simulink model "TV_full_CARSIM_24b"  (R2024b)
settings: Solver=FixedStepAuto  StartTime=0  StopTime=30  FixedStep=0.0005  RelTol=1e-3
undefined symbols (not defined in the file): DGain, FBgain, FFgain, g, GR, h, IGain, Iz, Kb, Kd, Ki, Kn, Kp, L, mu, Mz_dTm_convertion, NGain, PGain, s_desired, TC_switch, Tmax, TV_switch, vx_vector
libraries: slpidlib x2, Solver_SF x1, simulink x1
settings Model: Creator=savchenko.6  LastModifiedBy=account
settings DataIOCC: ReturnWorkspaceOutputs=off
settings RTWCC: GPUComputeCapability=3.5
settings ConfigComp: CovBoundaryAbsTol=1.0e-5

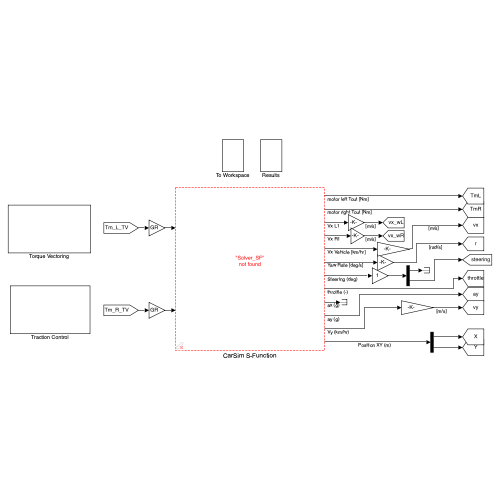
[thumbnail: Simulink's stored preview of the top-level diagram]
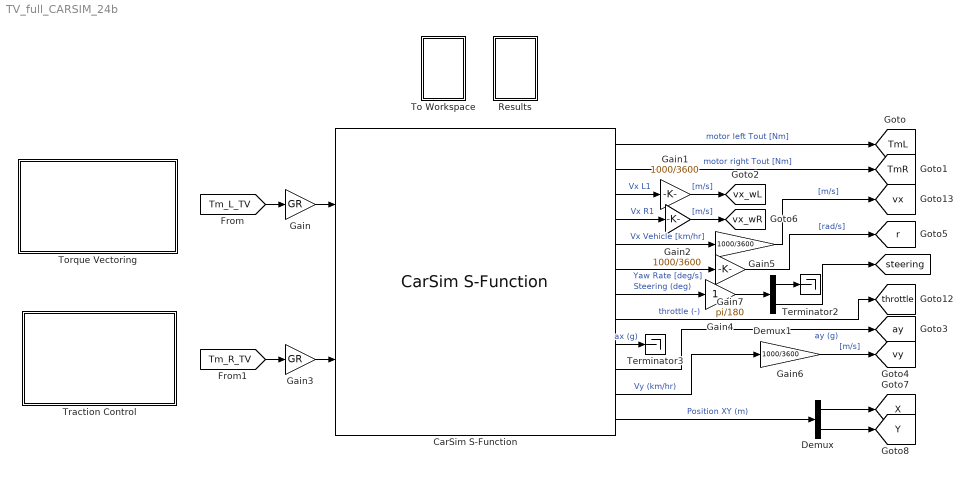
== system TV_full_CARSIM_24b ==
  CarSim S-Function : Solver_SF/CarSim S-Function  Priority=1  SIMFILE=simfile.sim  Run_RTs=off  vs_state_ind=Run  StopMode_ind=Vehicle Model
  Demux : Demux  Outputs=2
  Demux1 : Demux  Outputs=2
  Gain : Gain  Gain=GR
  Gain{1..2,5..6} (4 alike) : Gain  Gain=1000/3600
  Gain3 : Gain  Gain=GR
  Gain4 : Gain
  Gain7 : Gain  Gain=pi/180
  Results : Subsystem
  Terminator2 : Terminator
  Terminator3 : Terminator
  To Workspace : Subsystem
  Torque Vectoring : Subsystem
  Traction Control : Subsystem
  tag scope: TmL=global, TmR=global, X=global, Y=global, ay=global, r=global, steering=global, throttle=global, vx=global, vx_wL=global, vx_wR=global, vy=global
  wires:
  CarSim S-Function/5 -> Gain5/1  "Vx Vehicle [km/hr]"
  CarSim S-Function/10 -> [ay]  "ay (g)"
  CarSim S-Function/11 -> Gain6/1  "Vy (km/hr)"
  CarSim S-Function/6 -> Gain7/1  "Yaw Rate [deg/s]"
  CarSim S-Function/1 -> [TmL]  "motor left Tout [Nm]"
  CarSim S-Function/2 -> [TmR]  "motor right Tout [Nm]"
  CarSim S-Function/3 -> Gain1/1  "Vx L1"
  CarSim S-Function/4 -> Gain2/1  "Vx R1"
  CarSim S-Function/7 -> Gain4/1  "Steering (deg)"
  CarSim S-Function/8 -> [throttle]  "throttle (-)"
  CarSim S-Function/9 -> Terminator3/1  "ax (g)"
  CarSim S-Function/12 -> Demux/1  "Position XY (m)"
  Demux/1 -> [X]
  Demux/2 -> [Y]
  Gain7/1 -> [r]  "[rad/s]"
  Gain5/1 -> [vx]  "[m/s]"
  Demux1/1 -> Terminator2/1
  Gain1/1 -> [vx_wL]  "[m/s]"
  Gain2/1 -> [vx_wR]  "[m/s]"
  [Tm_R_TV] -> Gain3/1
  [Tm_L_TV] -> Gain/1
  Gain/1 -> CarSim S-Function/1
  Gain3/1 -> CarSim S-Function/2
  Gain4/1 -> Demux1/1
  Gain6/1 -> [vy]  "[m/s]"
  Demux1/2 -> [steering]

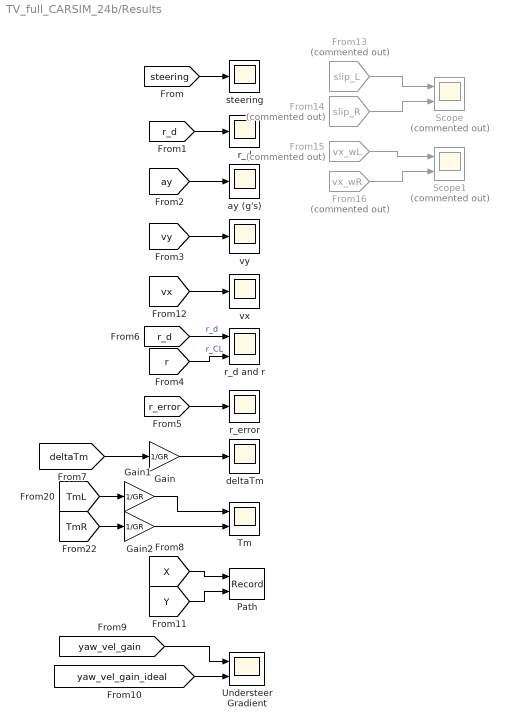
== system TV_full_CARSIM_24b/Results ==
  From13 : From  Commented=on  GotoTag=slip_L  TagVisibility=global
  From14 : From  Commented=on  GotoTag=slip_R  TagVisibility=global
  From15 : From  Commented=on  GotoTag=vx_wL  TagVisibility=global
  From16 : From  Commented=on  GotoTag=vx_wR  TagVisibility=global
  Gain : Gain  Gain=1/GR
  Gain1 : Gain  Gain=1/GR
  Gain2 : Gain  Gain=1/GR
  Path : Record  FileSettingsInternal="{\"entries\":[{\"content\":{\"excelSettings\":{\"content\":{},\"type\":\"Streamout.ExcelSettings\"},\"parquetSettings\":{\"content\":{},\"type\":\"Streamout.ParquetSettings\"}},\"type\":\"Streamout.FileSettingStorage\",\"uuid\":\"\"}],\"packageUris\":[\"http:\\/\\/schema.mathworks.com\\/mf0\\/streamout_blocks\\/R2020a\"],\"version\":\"1.0\"}"  Layout=[1 1]  SignalsInternal="{\"entries\":[{\"content\":{\"signals\":[{\"content\":{\"blockPath\":[],\"dimensions\":[1],\"domain\":\"\",\"lineColor\":\"#fe330a\",\"port\":1,\"signalID\":1,\"signalName\":\"From8\"},\"type\":\"RecordBlkView.Signal\",\"uuid\":\"\"},{\"content\":{\"blockPath\":[],\"dimensions\":[1],\"domain\":\"\",\"lineColor\":\"#22b573\",\"port\":2,\"signalID\":2,\"signalName\":\"From11\"},\"type\":\"RecordBlkView.Signal\",\"uuid\":\"\"}]},\"type\":\"RecordBlkView.InputSignals\",\"uuid\":\"\"}],\"packageUris\":[\"http:\\/\\/schema.mathworks.com\\/mf0\\/streamout_blocks\\/R2020a\"],\"version\":\"1.0\"}"  VisualizationBindings="{\"xyplotplugin\":{\"info\":[{\"series\":[],\"subplotID\":1}]}}"  CompatibilityTag=XY
  Scope : Scope  Commented=on  NumInputPorts=2
  Scope1 : Scope  Commented=on  NumInputPorts=2
  Tm : Scope  NumInputPorts=2
  Understeer Gradient : Scope  NumInputPorts=2
  ay (g's) : Scope
  deltaTm : Scope
  r_d : Scope
  r_d and r : Scope  NumInputPorts=2
  r_error : Scope
  steering : Scope
  vx : Scope
  vy : Scope
  wires:
  [deltaTm] -> Gain/1
  [r] -> r_d and r/2  "r_CL"
  [TmR] -> Gain2/1
  [steering] -> steering/1
  [Y] -> Path/2
  [vy] -> vy/1
  [TmL] -> Gain1/1
  [r_d] -> r_d and r/1  "r_d"
  [r_d] -> r_d/1
  [ay] -> ay (g's)/1
  [r_error] -> r_error/1
  [X] -> Path/1
  [yaw_vel_gain] -> Understeer Gradient/1
  [yaw_vel_gain_ideal] -> Understeer Gradient/2
  [vx] -> vx/1
  From13/1 -> Scope/1
  From14/1 -> Scope/2
  From15/1 -> Scope1/1
  From16/1 -> Scope1/2
  Gain/1 -> deltaTm/1
  Gain1/1 -> Tm/1
  Gain2/1 -> Tm/2

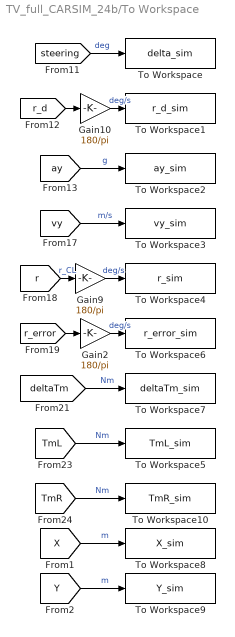
== system TV_full_CARSIM_24b/To Workspace ==
  Gain10 : Gain  Gain=180/pi
  Gain2 : Gain  Gain=180/pi
  Gain9 : Gain  Gain=180/pi
  To Workspace : ToWorkspace  VariableName=delta_sim  SampleTime=-1
  To Workspace1 : ToWorkspace  VariableName=r_d_sim  SampleTime=-1
  To Workspace10 : ToWorkspace  VariableName=TmR_sim  SampleTime=-1
  To Workspace2 : ToWorkspace  VariableName=ay_sim  SampleTime=-1
  To Workspace3 : ToWorkspace  VariableName=vy_sim  SampleTime=-1
  To Workspace4 : ToWorkspace  VariableName=r_sim  SampleTime=-1
  To Workspace5 : ToWorkspace  VariableName=TmL_sim  SampleTime=-1
  To Workspace6 : ToWorkspace  VariableName=r_error_sim  SampleTime=-1
  To Workspace7 : ToWorkspace  VariableName=deltaTm_sim  SampleTime=-1
  To Workspace8 : ToWorkspace  VariableName=X_sim  SampleTime=-1
  To Workspace9 : ToWorkspace  VariableName=Y_sim  SampleTime=-1
  wires:
  [vy] -> To Workspace3/1  "m/s"
  [ay] -> To Workspace2/1  "g"
  Gain10/1 -> To Workspace1/1  "deg/s"
  [deltaTm] -> To Workspace7/1  "Nm"
  Gain2/1 -> To Workspace6/1  "deg/s"
  [TmR] -> To Workspace10/1  "Nm"
  [r] -> Gain9/1  "r_CL"
  [steering] -> To Workspace/1  "deg"
  [r_d] -> Gain10/1
  [TmL] -> To Workspace5/1  "Nm"
  [r_error] -> Gain2/1
  Gain9/1 -> To Workspace4/1  "deg/s"
  [X] -> To Workspace8/1  "m"
  [Y] -> To Workspace9/1  "m"

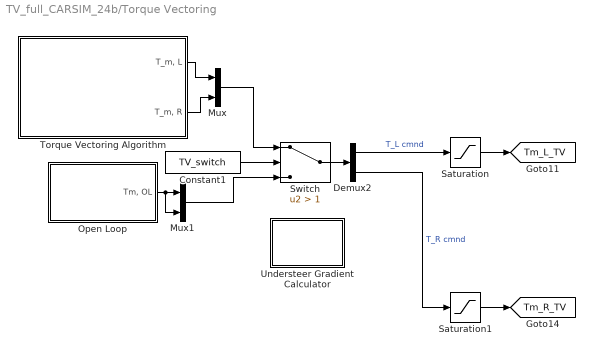
== system TV_full_CARSIM_24b/Torque Vectoring ==
  Constant1 : Constant  Value=TV_switch
  Demux2 : Demux  Outputs=2
  Mux : Mux  Inputs=2
  Mux1 : Mux  Inputs=2
  Open Loop : Subsystem
  Saturation : Saturate  UpperLimit=Tmax  LowerLimit=0
  Saturation1 : Saturate  UpperLimit=Tmax  LowerLimit=0
  Switch : Switch  Criteria=u2 > Threshold  Threshold=1  SaturateOnIntegerOverflow=off  InputSameDT=off
  Torque Vectoring Algorithm : Subsystem
  Understeer Gradient Calculator : Subsystem
  tag scope: Tm_L_TV=global, Tm_R_TV=global
  wires:
  Demux2/2 -> Saturation1/1  "T_R cmnd"
  Mux/1 -> Switch/1
  Constant1/1 -> Switch/2
  Torque Vectoring Algorithm/2("T_m, R") -> Mux/2
  Demux2/1 -> Saturation/1  "T_L cmnd"
  Open Loop/1("Tm, OL") -> Mux1/2, Mux1/1
  Torque Vectoring Algorithm/1("T_m, L") -> Mux/1
  Mux1/1 -> Switch/3
  Switch/1 -> Demux2/1
  Saturation/1 -> [Tm_L_TV]
  Saturation1/1 -> [Tm_R_TV]

== system TV_full_CARSIM_24b/Traction Control ==
  Trcation Control Algorithm : Subsystem
  tag scope: Tm_L_TC=global, Tm_R_TC=global, slip=global, slip_L=global, slip_R=global
  wires:
  [Tm_R_TV] -> Trcation Control Algorithm/5(Tm_R_TV)
  Trcation Control Algorithm/3(Tm_R_TC) -> [Tm_R_TC]
  [vx_wL] -> Trcation Control Algorithm/2(vx_wL)
  Trcation Control Algorithm/1(slip_L) -> [slip_L]
  Trcation Control Algorithm/4(Tm_L_TC) -> [Tm_L_TC]
  Trcation Control Algorithm/2(slip_R) -> [slip_R]
  [Tm_L_TV] -> Trcation Control Algorithm/4(Tm_L_TV)
  [vx_wR] -> Trcation Control Algorithm/3(vx_wR)
  [vx] -> Trcation Control Algorithm/1(vx)
  Trcation Control Algorithm/5(slip) -> [slip]

== system TV_full_CARSIM_24b/Torque Vectoring/Open Loop ==
  Gain : Gain  Gain=21
  "Tm, OL" : Outport
  wires:
  [throttle] -> Gain/1
  Gain/1 -> "Tm, OL"/1

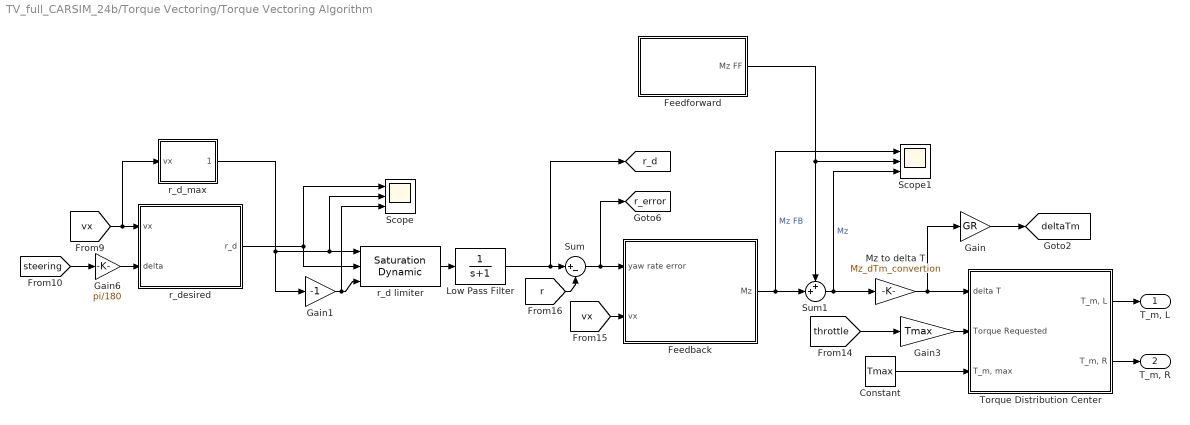
== system TV_full_CARSIM_24b/Torque Vectoring/Torque Vectoring Algorithm ==
  Constant : Constant  Value=Tmax
  Feedback : Subsystem
  Feedforward : Subsystem
  Gain : Gain  Gain=GR
  Gain1 : Gain  Gain=-1
  Gain3 : Gain  Gain=Tmax
  Gain6 : Gain  Gain=pi/180
  Low Pass Filter : TransferFcn  Denominator=[1 1]
  Mz to delta T : Gain  Gain=Mz_dTm_convertion
  Scope : Scope  NumInputPorts=3
  Scope1 : Scope  NumInputPorts=3
  Sum : Sum  Inputs=|+-
  Sum1 : Sum  Inputs=++|
  Torque Distribution Center : Subsystem
  r_d limiter : simulink/Discontinuities/Saturation Dynamic  OutMin=[]  OutMax=[]  OutDataTypeStr=Inherit: Same as second input  OutDataType=fixdt(1, 16)  OutScaling=2^-10  RndMeth=Round  DoSatur=off
  r_d_max : Subsystem
  r_desired : Subsystem
  "T_m, L" : Outport
  "T_m, R" : Outport  Port=2
  tag scope: deltaTm=global, r_d=global, r_error=global
  wires:
  r_d_max/1(r_d_max) -> Scope/2, r_d limiter/1, Gain1/1
  Sum/1 -> Feedback/1(yaw rate error), [r_error]
  r_desired/1(r_d) -> r_d limiter/2, Scope/1
  Gain3/1 -> Torque Distribution Center/2(Torque Requested)
  [r] -> Sum/2
  [steering] -> Gain6/1
  Gain1/1 -> Scope/3, r_d limiter/3
  [throttle] -> Gain3/1
  [vx] -> r_d_max/1(vx), r_desired/1(vx)
  Mz to delta T/1 -> Torque Distribution Center/1(delta T), Gain/1
  Gain6/1 -> r_desired/2(delta)
  Constant/1 -> Torque Distribution Center/3("T_m, max")
  [vx] -> Feedback/2(vx)
  Feedback/1(Mz) -> Scope1/1, Sum1/2  "Mz FB"
  Sum1/1 -> Scope1/3, Mz to delta T/1  "Mz"
  r_d limiter/1 -> Low Pass Filter/1
  Low Pass Filter/1 -> [r_d], Sum/1
  Feedforward/1(Mz FF) -> Sum1/1, Scope1/2
  Torque Distribution Center/1("T_m, L") -> "T_m, L"/1
  Torque Distribution Center/2("T_m, R") -> "T_m, R"/1
  Gain/1 -> [deltaTm]

== system TV_full_CARSIM_24b/Torque Vectoring/Understeer Gradient Calculator ==
  To Workspace1 : ToWorkspace  VariableName=yaw_vel_gain  SampleTime=-1
  To Workspace2 : ToWorkspace  VariableName=ideal_yaw_vel_gain  SampleTime=-1
  When velocity is >0 : Subsystem  TreatAsAtomicUnit=on
  tag scope: yaw_vel_gain=global, yaw_vel_gain_ideal=global
  wires:
  [vx] -> When velocity is >0/Enable, When velocity is >0/3(Vx)
  [r] -> When velocity is >0/1(r)
  When velocity is >0/2(ideal yaw velocity gain) -> [yaw_vel_gain_ideal], To Workspace2/1  "ideal"
  When velocity is >0/1(yaw velocity gain) -> [yaw_vel_gain], To Workspace1/1  "actual"
  [steering] -> When velocity is >0/2(delta_f)

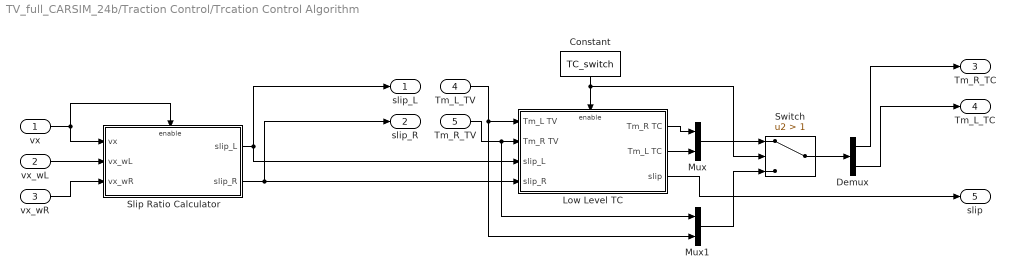
== system TV_full_CARSIM_24b/Traction Control/Trcation Control Algorithm ==
  vx : Inport
  vx_wL : Inport  Port=2
  vx_wR : Inport  Port=3
  Tm_L_TV : Inport  Port=4
  Tm_R_TV : Inport  Port=5
  Constant : Constant  Value=TC_switch
  Demux : Demux  Outputs=2
  Low Level TC : Subsystem
  Mux : Mux  Inputs=2
  Mux1 : Mux  Inputs=2
  Slip Ratio Calculator : Subsystem
  Switch : Switch  Criteria=u2 > Threshold  Threshold=1  SaturateOnIntegerOverflow=off  InputSameDT=off
  slip_L : Outport
  slip_R : Outport  Port=2
  Tm_R_TC : Outport  Port=3
  Tm_L_TC : Outport  Port=4
  slip : Outport  Port=5
  wires:
  Slip Ratio Calculator/2(slip_R) -> slip_R/1, Low Level TC/4(slip_R)
  Slip Ratio Calculator/1(slip_L) -> slip_L/1, Low Level TC/3(slip_L)
  vx_wL/1 -> Slip Ratio Calculator/2(vx_wL)
  vx/1 -> Slip Ratio Calculator/Enable, Slip Ratio Calculator/1(vx)
  vx_wR/1 -> Slip Ratio Calculator/3(vx_wR)
  Tm_L_TV/1 -> Mux1/2, Low Level TC/1(Tm_L TV)
  Tm_R_TV/1 -> Mux1/1, Low Level TC/2(Tm_R TV)
  Low Level TC/1(Tm_R TC) -> Mux/1
  Low Level TC/2(Tm_L TC) -> Mux/2
  Mux/1 -> Switch/1
  Mux1/1 -> Switch/3
  Switch/1 -> Demux/1
  Demux/1 -> Tm_R_TC/1
  Demux/2 -> Tm_L_TC/1
  Constant/1 -> Switch/2, Low Level TC/Enable
  Low Level TC/3(slip) -> slip/1

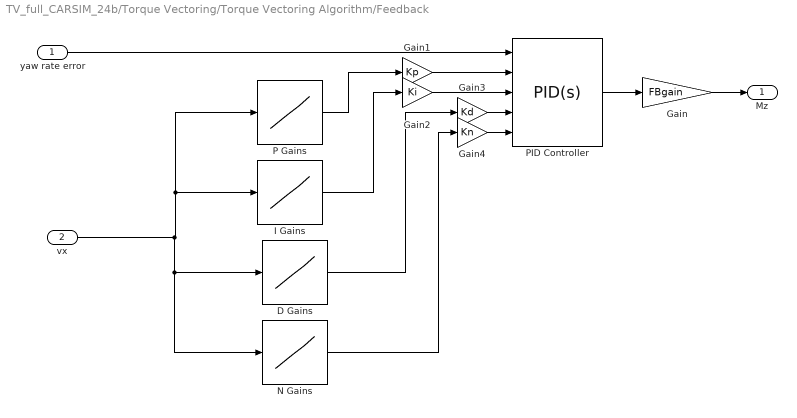
== system TV_full_CARSIM_24b/Torque Vectoring/Torque Vectoring Algorithm/Feedback ==
  yaw rate error : Inport
  vx : Inport  Port=2
  D Gains : Lookup_n-D  NumberOfTableDimensions=1  LookupTableObject=''  BreakpointsForDimension1=vx_vector  BreakpointsForDimension1FirstPoint=10  BreakpointsForDimension2FirstPoint=10  BreakpointsForDimension1Spacing=12  BreakpointsForDimension2Spacing=12  IndexSearchMethod=Evenly spaced points  Table=DGain  RemoveProtectionInput=on  InternalRulePriority=Speed  RndMeth=Simplest
  Gain : Gain  Gain=FBgain
  Gain1 : Gain  Gain=Kp
  Gain2 : Gain  Gain=Ki
  Gain3 : Gain  Gain=Kd
  Gain4 : Gain  Gain=Kn
  I Gains : Lookup_n-D  NumberOfTableDimensions=1  LookupTableObject=''  BreakpointsForDimension1=vx_vector  BreakpointsForDimension1FirstPoint=10  BreakpointsForDimension2FirstPoint=10  BreakpointsForDimension1Spacing=12  BreakpointsForDimension2Spacing=12  IndexSearchMethod=Evenly spaced points  Table=IGain  RemoveProtectionInput=on  InternalRulePriority=Speed  RndMeth=Simplest
  N Gains : Lookup_n-D  NumberOfTableDimensions=1  LookupTableObject=''  BreakpointsForDimension1=vx_vector  BreakpointsForDimension1FirstPoint=10  BreakpointsForDimension2FirstPoint=10  BreakpointsForDimension1Spacing=12  BreakpointsForDimension2Spacing=12  IndexSearchMethod=Evenly spaced points  Table=NGain  RemoveProtectionInput=on  InternalRulePriority=Speed  RndMeth=Simplest
  P Gains : Lookup_n-D  NumberOfTableDimensions=1  LookupTableObject=''  BreakpointsForDimension1=vx_vector  BreakpointsForDimension1FirstPoint=10  BreakpointsForDimension2FirstPoint=10  BreakpointsForDimension1Spacing=12  BreakpointsForDimension2Spacing=12  IndexSearchMethod=Evenly spaced points  Table=PGain  RemoveProtectionInput=on  InternalRulePriority=Speed  RndMeth=Simplest
  PID Controller : slpidlib/PID Controller  Controller=PID  Form=Parallel  TimeDomain=Continuous-time  UseExternalTs=off  SampleTime=-1  IntegratorMethod=Forward Euler  FilterMethod=Forward Euler  ControllerParametersSource=external  P=122.511124072632  I=58.1909076470783  UseKiTs=off  D=21.7107369694367  UseExternalDerivativeSource=off  N=2  UseFilter=on  TunerSelectOption=Transfer Function Based (PID Tuner App)  InitialConditionSource=internal  InitialConditionForIntegrator=0  InitialConditionForFilter=0  DifferentiatorICPrevScaledInput=0  ExternalReset=none  TrackingMode=off  Kt=1  LimitOutput=on  SatLimitsSource=internal  UpperSaturationLimit=10  LowerSaturationLimit=-10  LinearizeAsGain=on  AntiWindupMode=back-calculation  Kb=Kb  LimitIntegrator=off  UpperIntegratorSaturationLimit=inf  LowerIntegratorSaturationLimit=-inf  POutMin=[]  POutMax=[]  IOutMin=[]  IOutMax=[]  DOutMin=[]  DOutMax=[]  NOutMin=[]  NOutMax=[]  SumOutMin=[]  SumOutMax=[]  SaturationOutMin=[]  SaturationOutMax=[]  PParamMin=[]  PParamMax=[]  IParamMin=[]  IParamMax=[]  DParamMin=[]  DParamMax=[]  NParamMin=[]  NParamMax=[]  KbParamMin=[]  KbParamMax=[]  KtParamMin=[]  KtParamMax=[]  KbOutMin=[]  KbOutMax=[]  KtOutMin=[]  KtOutMax=[]  IntegratorOutMin=[]  IntegratorOutMax=[]  FilterOutMin=[]  FilterOutMax=[]  SumI1OutMin=[]  SumI1OutMax=[]  SumI2OutMin=[]  SumI2OutMax=[]  SumI3OutMin=[]  SumI3OutMax=[]  SumI4OutMin=[]  SumI4OutMax=[]  SumDOutMin=[]  SumDOutMax=[]  DifferentiatorOutMin=[]  DifferentiatorOutMax=[]  FilterDiffOutCoefMin=[]  FilterDiffOutCoefMax=[]  ReciprocalOutMin=[]  ReciprocalOutMax=[]  SumDenOutMin=[]  SumDenOutMax=[]  SumNumOutMin=[]  SumNumOutMax=[]  DivideOutMin=[]  DivideOutMax=[]  UdiffTsProdOutMin=[]  UdiffTsProdOutMax=[]  NTsProdOutMin=[]  NTsProdOutMax=[]  UintegralTsProdOutMin=[]  UintegralTsProdOutMax=[]  UngainTsProdOutMin=[]  UngainTsProdOutMax=[]  ClampingZeroOutDataTypeStr=Inherit: Inherit via back propagation  ClampingZeroOutMin=[]  ClampingZeroOutMax=[]  FilterDenConstantOutDataTypeStr=Inherit: Inherit via back propagation  FilterDenConstantOutMin=[]  FilterDenConstantOutMax=[]  PCopyOutDataTypeStr=Inherit: Inherit via back propagation  PCopyOutMin=[]  PCopyOutMax=[]  NCopyOutDataTypeStr=Inherit: Inherit via back propagation  NCopyOutMin=[]  NCopyOutMax=[]  IntegratorContinuousStateAttributes=''  IntegratorStateMustResolveToSignalObject=off  IntegratorRTWStateStorageClass=Auto  FilterContinuousStateAttributes=''  FilterStateMustResolveToSignalObject=off  FilterRTWStateStorageClass=Auto  ParallelPVariant=ExternalParameters  IdealPVariant=Disabled  IVariant=ExternalParameters  DVariant=ExternalParameters  IntegratorVariant=Continuous  SatVariant=Enabled  AWVariant=BackCalculation  PCopyVariant=Disabled  TRVariant=Disabled  FdbkBlocksVariant=Forward  IdealPFdbkVariant=Disabled  SatFdbkVariant=Disabled  DerivativeFilterVariant=ContFilter  NVariant=ExternalParameters  NCopyVariant=Disabled  FilterICVariant=InternalICsFilter  IntegratorICVariant=InternalICs  ExternalResetVariant=Disabled  TRSumVariant=Passthrough  SumFdbkVariant=Disabled  SumVariant=Sum_PID  TsampFilterVariant=InternalTs  TsampNgainVariant=Passthrough  TsampIntegralVariant=Disabled_SignalSpec  ExternalSaturationOutDataTypeStr=Inherit: Same as second input  DerivativeSourceVariant=ErrorSignal  PreIntVariant=InternalPreInt
  Mz : Outport
  wires:
  yaw rate error/1 -> PID Controller/1
  vx/1 -> N Gains/1, D Gains/1, I Gains/1, P Gains/1
  I Gains/1 -> Gain2/1
  N Gains/1 -> Gain4/1
  PID Controller/1 -> Gain/1
  Gain/1 -> Mz/1
  P Gains/1 -> Gain1/1
  D Gains/1 -> Gain3/1
  Gain1/1 -> PID Controller/2
  Gain2/1 -> PID Controller/3
  Gain3/1 -> PID Controller/4
  Gain4/1 -> PID Controller/5

== system TV_full_CARSIM_24b/Torque Vectoring/Torque Vectoring Algorithm/Feedforward ==
  Gain : Gain  Gain=Iz
  Gain2 : Gain  Gain=FFgain
  Mz FF : Outport
  wires:
  [r_d] -> Gain/1
  Gain/1 -> Gain2/1
  Gain2/1 -> Mz FF/1  "Mz FF"

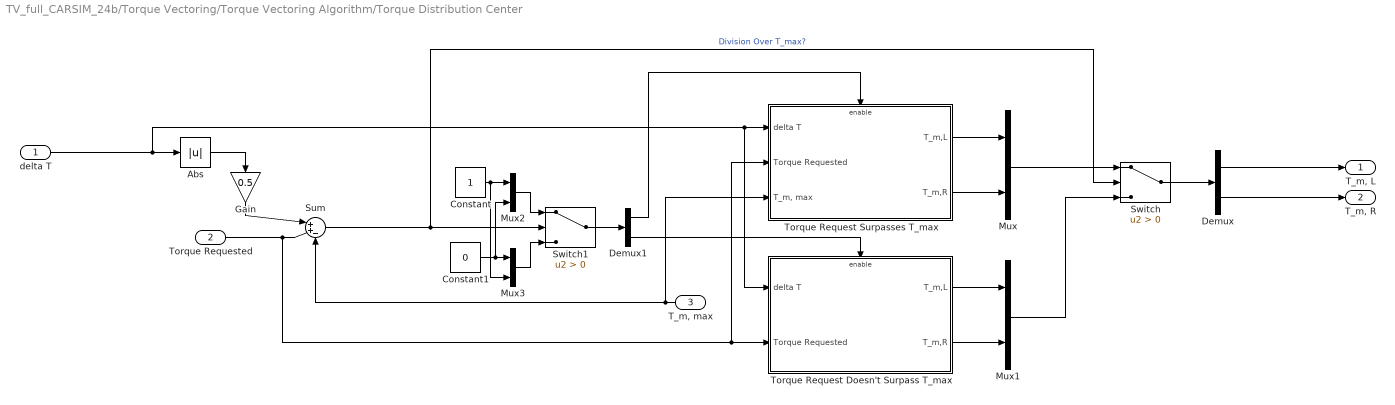
== system TV_full_CARSIM_24b/Torque Vectoring/Torque Vectoring Algorithm/Torque Distribution Center ==
  delta T : Inport
  Torque Requested : Inport  Port=2
  "T_m, max" : Inport  Port=3
  Abs : Abs  SaturateOnIntegerOverflow=off
  Constant : Constant
  Constant1 : Constant  Value=0
  Demux : Demux  Outputs=2
  Demux1 : Demux  Outputs=2
  Gain : Gain  Gain=0.5
  Mux{,1..3} (4 alike) : Mux  Inputs=2
  Sum : Sum  Inputs=|++-
  Switch : Switch  Criteria=u2 > Threshold  SaturateOnIntegerOverflow=off  InputSameDT=off
  Switch1 : Switch  Criteria=u2 > Threshold  SaturateOnIntegerOverflow=off  InputSameDT=off
  Torque Request Doesn't Surpass T_max : Subsystem  TreatAsAtomicUnit=on
  Torque Request Surpasses T_max : Subsystem  TreatAsAtomicUnit=on
  "T_m, L" : Outport
  "T_m, R" : Outport  Port=2
  wires:
  Sum/1 -> Switch1/2, Switch/2  "Division Over T_max?"
  Gain/1 -> Sum/1
  Abs/1 -> Gain/1
  Torque Request Surpasses T_max/1(T_m,L) -> Mux/1
  Torque Request Surpasses T_max/2(T_m,R) -> Mux/2
  Torque Request Doesn't Surpass T_max/1(T_m,L) -> Mux1/1
  Torque Request Doesn't Surpass T_max/2(T_m,R) -> Mux1/2
  Mux/1 -> Switch/1
  Mux1/1 -> Switch/3
  Switch/1 -> Demux/1
  Torque Requested/1 -> Torque Request Surpasses T_max/2(Torque Requested), Torque Request Doesn't Surpass T_max/2(Torque Requested), Sum/2
  "T_m, max"/1 -> Sum/3, Torque Request Surpasses T_max/3("T_m, max")
  Mux2/1 -> Switch1/1
  Mux3/1 -> Switch1/3
  Switch1/1 -> Demux1/1
  Demux1/1 -> Torque Request Surpasses T_max/Enable
  Demux1/2 -> Torque Request Doesn't Surpass T_max/Enable
  Constant/1 -> Mux2/1, Mux3/2
  Constant1/1 -> Mux2/2, Mux3/1
  delta T/1 -> Torque Request Doesn't Surpass T_max/1(delta T), Torque Request Surpasses T_max/1(delta T), Abs/1
  Demux/1 -> "T_m, L"/1
  Demux/2 -> "T_m, R"/1

== system TV_full_CARSIM_24b/Torque Vectoring/Torque Vectoring Algorithm/r_d_max ==
  vx : Inport
  Constant : Constant  Value=0.85*mu*g/(1+(h/t))
  Divide : Product  Inputs=*/
  Saturation : Saturate  UpperLimit=1000000  LowerLimit=0.01
  r_d_max : Outport
  wires:
  Constant/1 -> Divide/1
  vx/1 -> Saturation/1
  Saturation/1 -> Divide/2
  Divide/1 -> r_d_max/1

== system TV_full_CARSIM_24b/Torque Vectoring/Torque Vectoring Algorithm/r_desired ==
  vx : Inport
  delta : Inport  Port=2
  Gain : Gain  Gain=1/L
  Product : Product
  Tan : Trigonometry  Operator=tan
  r_d : Outport
  wires:
  delta/1 -> Tan/1
  vx/1 -> Product/1
  Tan/1 -> Product/2
  Product/1 -> Gain/1
  Gain/1 -> r_d/1

== system TV_full_CARSIM_24b/Torque Vectoring/Understeer Gradient Calculator/When velocity is >0 ==
  r : Inport
  delta_f : Inport  Port=2
  Vx : Inport  Port=3
  Enable : EnablePort  StatesWhenEnabling=reset
  Gain : Gain  Gain=1/L
  When Steering : Subsystem  TreatAsAtomicUnit=on
  deg to rad : Gain  Gain=pi/180
  yaw velocity gain : Outport
  ideal yaw velocity gain : Outport  Port=2
  wires:
  delta_f/1 -> deg to rad/1
  r/1 -> When Steering/1(r)
  When Steering/1(yaw velocity gain) -> yaw velocity gain/1
  deg to rad/1 -> When Steering/2(delta_f), When Steering/Enable
  Vx/1 -> Gain/1
  Gain/1 -> ideal yaw velocity gain/1

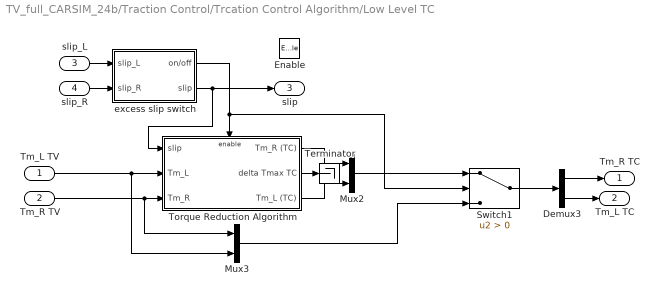
== system TV_full_CARSIM_24b/Traction Control/Trcation Control Algorithm/Low Level TC ==
  Tm_L TV : Inport
  Tm_R TV : Inport  Port=2
  slip_L : Inport  Port=3
  slip_R : Inport  Port=4
  Enable : EnablePort
  Demux3 : Demux  Outputs=2
  Mux2 : Mux  Inputs=2
  Mux3 : Mux  Inputs=2
  Switch1 : Switch  Criteria=u2 > Threshold  SaturateOnIntegerOverflow=off  InputSameDT=off
  Terminator : Terminator
  Torque Reduction Algorithm : Subsystem  TreatAsAtomicUnit=on
  excess slip switch : Subsystem
  Tm_R TC : Outport
  Tm_L TC : Outport  Port=2
  slip : Outport  Port=3
  wires:
  Demux3/2 -> Tm_L TC/1
  Mux3/1 -> Switch1/3
  Tm_L TV/1 -> Mux3/2, Torque Reduction Algorithm/2(Tm_L)
  Torque Reduction Algorithm/2(delta Tmax TC) -> Terminator/1
  Tm_R TV/1 -> Mux3/1, Torque Reduction Algorithm/3(Tm_R)
  Torque Reduction Algorithm/1(Tm_R (TC)) -> Mux2/1
  excess slip switch/1(on/off) -> Switch1/2, Torque Reduction Algorithm/Enable
  Mux2/1 -> Switch1/1
  Torque Reduction Algorithm/3(Tm_L (TC)) -> Mux2/2
  Switch1/1 -> Demux3/1
  Demux3/1 -> Tm_R TC/1
  excess slip switch/2(slip) -> Torque Reduction Algorithm/1(slip), slip/1
  slip_L/1 -> excess slip switch/1(slip_L)
  slip_R/1 -> excess slip switch/2(slip_R)

== system TV_full_CARSIM_24b/Traction Control/Trcation Control Algorithm/Slip Ratio Calculator ==
  vx : Inport
  vx_wL : Inport  Port=2
  vx_wR : Inport  Port=3
  Enable : EnablePort
  Divide : Product  Inputs=*/
  Divide1 : Product  Inputs=*/
  Subtract : Sum  Inputs=+-
  Subtract1 : Sum  Inputs=+-
  slip_L : Outport
  slip_R : Outport  Port=2
  wires:
  Subtract/1 -> Divide/1
  vx/1 -> Subtract1/1, Divide/2, Divide1/2, Subtract/1
  Divide/1 -> slip_L/1
  Divide1/1 -> slip_R/1
  Subtract1/1 -> Divide1/1
  vx_wR/1 -> Subtract1/2
  vx_wL/1 -> Subtract/2

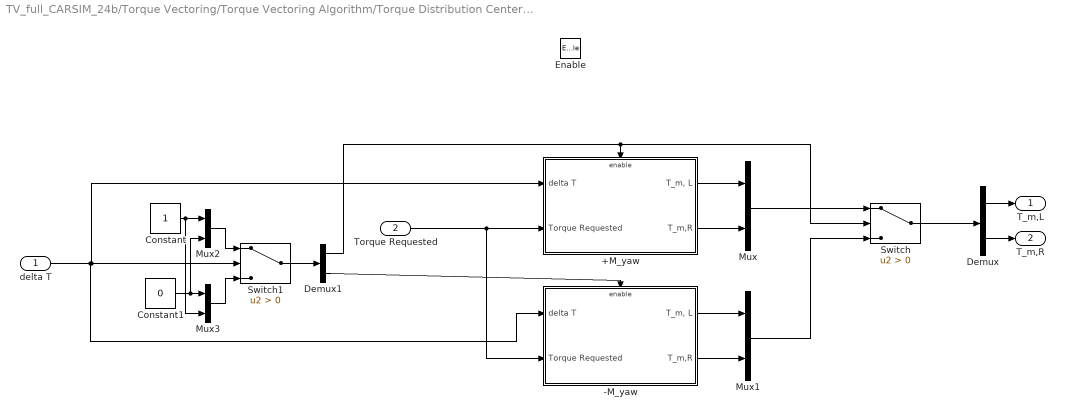
== system TV_full_CARSIM_24b/Torque Vectoring/Torque Vectoring Algorithm/Torque Distribution Center/Torque Request Doesn't Surpass T_max ==
  delta T : Inport
  Torque Requested : Inport  Port=2
  Enable : EnablePort  StatesWhenEnabling=reset
  +M_yaw : Subsystem  TreatAsAtomicUnit=on
  -M_yaw : Subsystem  TreatAsAtomicUnit=on
  Constant : Constant
  Constant1 : Constant  Value=0
  Demux : Demux  Outputs=2
  Demux1 : Demux  Outputs=2
  Mux{,1..3} (4 alike) : Mux  Inputs=2
  Switch : Switch  Criteria=u2 > Threshold  SaturateOnIntegerOverflow=off  InputSameDT=off
  Switch1 : Switch  Criteria=u2 > Threshold  SaturateOnIntegerOverflow=off  InputSameDT=off
  T_m,L : Outport
  T_m,R : Outport  Port=2
  wires:
  +M_yaw/1("T_m, L") -> Mux/1
  +M_yaw/2(T_m,R) -> Mux/2
  -M_yaw/1("T_m, L") -> Mux1/1
  -M_yaw/2(T_m,R) -> Mux1/2
  Mux/1 -> Switch/1
  Mux1/1 -> Switch/3
  Torque Requested/1 -> -M_yaw/2(Torque Requested), +M_yaw/2(Torque Requested)
  Switch/1 -> Demux/1
  Demux/1 -> T_m,L/1
  Demux/2 -> T_m,R/1
  Mux2/1 -> Switch1/1
  Demux1/1 -> Switch/2, +M_yaw/Enable
  Demux1/2 -> -M_yaw/Enable
  Mux3/1 -> Switch1/3
  Switch1/1 -> Demux1/1
  Constant1/1 -> Mux2/2, Mux3/1
  Constant/1 -> Mux2/1, Mux3/2
  delta T/1 -> Switch1/2, +M_yaw/1(delta T), -M_yaw/1(delta T)

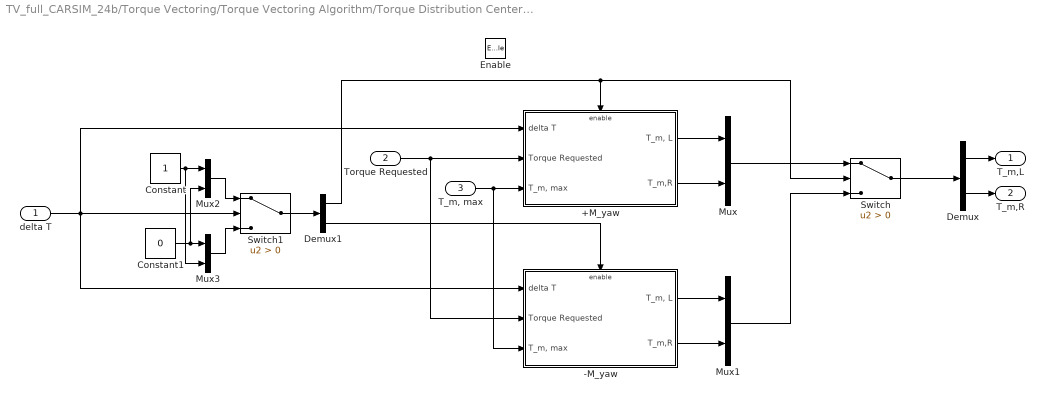
== system TV_full_CARSIM_24b/Torque Vectoring/Torque Vectoring Algorithm/Torque Distribution Center/Torque Request Surpasses T_max ==
  delta T : Inport
  Torque Requested : Inport  Port=2
  "T_m, max" : Inport  Port=3
  Enable : EnablePort  StatesWhenEnabling=reset
  +M_yaw : Subsystem  TreatAsAtomicUnit=on
  -M_yaw : Subsystem  TreatAsAtomicUnit=on
  Constant : Constant
  Constant1 : Constant  Value=0
  Demux : Demux  Outputs=2
  Demux1 : Demux  Outputs=2
  Mux{,1..3} (4 alike) : Mux  Inputs=2
  Switch : Switch  Criteria=u2 > Threshold  SaturateOnIntegerOverflow=off  InputSameDT=off
  Switch1 : Switch  Criteria=u2 > Threshold  SaturateOnIntegerOverflow=off  InputSameDT=off
  T_m,L : Outport
  T_m,R : Outport  Port=2
  wires:
  Mux/1 -> Switch/1
  Mux1/1 -> Switch/3
  Torque Requested/1 -> -M_yaw/2(Torque Requested), +M_yaw/2(Torque Requested)
  Demux/2 -> T_m,R/1
  Demux/1 -> T_m,L/1
  +M_yaw/2(T_m,R) -> Mux/2
  +M_yaw/1("T_m, L") -> Mux/1
  -M_yaw/2(T_m,R) -> Mux1/2
  Switch/1 -> Demux/1
  "T_m, max"/1 -> -M_yaw/3("T_m, max"), +M_yaw/3("T_m, max")
  -M_yaw/1("T_m, L") -> Mux1/1
  Mux2/1 -> Switch1/1
  Demux1/1 -> +M_yaw/Enable, Switch/2
  Demux1/2 -> -M_yaw/Enable
  Mux3/1 -> Switch1/3
  Switch1/1 -> Demux1/1
  Constant1/1 -> Mux2/2, Mux3/1
  Constant/1 -> Mux2/1, Mux3/2
  delta T/1 -> Switch1/2, -M_yaw/1(delta T), +M_yaw/1(delta T)

== system TV_full_CARSIM_24b/Torque Vectoring/Understeer Gradient Calculator/When velocity is >0/When Steering ==
  r : Inport
  delta_f : Inport  Port=2
  Enable : EnablePort  StatesWhenEnabling=reset
  Divide : Product  Inputs=*/
  yaw velocity gain : Outport
  wires:
  r/1 -> Divide/1
  delta_f/1 -> Divide/2
  Divide/1 -> yaw velocity gain/1

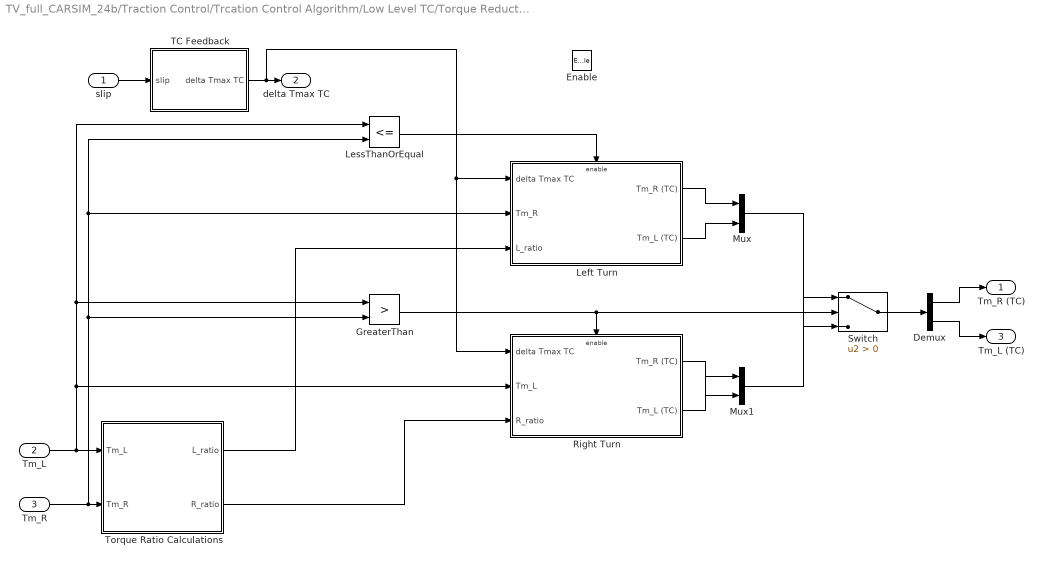
== system TV_full_CARSIM_24b/Traction Control/Trcation Control Algorithm/Low Level TC/Torque Reduction Algorithm ==
  slip : Inport
  Tm_L : Inport  Port=2
  Tm_R : Inport  Port=3
  Enable : EnablePort
  Demux : Demux  Outputs=2
  GreaterThan : RelationalOperator  Operator=>  OutDataTypeStr=boolean  RndMeth=Simplest  InputSameDT=off
  Left Turn : Subsystem  TreatAsAtomicUnit=on
  LessThanOrEqual : RelationalOperator  Operator=<=  OutDataTypeStr=boolean  RndMeth=Simplest  InputSameDT=off
  Mux : Mux  Inputs=2
  Mux1 : Mux  Inputs=2
  Right Turn : Subsystem  TreatAsAtomicUnit=on
  Switch : Switch  Criteria=u2 > Threshold  SaturateOnIntegerOverflow=off  InputSameDT=off
  TC Feedback : Subsystem
  Torque Ratio Calculations : Subsystem
  Tm_R (TC) : Outport
  delta Tmax TC : Outport  Port=2
  Tm_L (TC) : Outport  Port=3
  wires:
  Tm_L/1 -> GreaterThan/1, LessThanOrEqual/1, Right Turn/2(Tm_L), Torque Ratio Calculations/1(Tm_L)
  Tm_R/1 -> GreaterThan/2, LessThanOrEqual/2, Left Turn/2(Tm_R), Torque Ratio Calculations/2(Tm_R)
  LessThanOrEqual/1 -> Left Turn/Enable
  GreaterThan/1 -> Switch/2, Right Turn/Enable
  slip/1 -> TC Feedback/1(slip)
  TC Feedback/1(delta Tmax TC) -> Right Turn/1(delta Tmax TC), Left Turn/1(delta Tmax TC), delta Tmax TC/1
  Torque Ratio Calculations/1(L_ratio) -> Left Turn/3(L_ratio)
  Torque Ratio Calculations/2(R_ratio) -> Right Turn/3(R_ratio)
  Left Turn/1(Tm_R (TC)) -> Mux/1
  Left Turn/2(Tm_L (TC)) -> Mux/2
  Right Turn/2(Tm_L (TC)) -> Mux1/1
  Right Turn/1(Tm_R (TC)) -> Mux1/2
  Mux/1 -> Switch/3
  Mux1/1 -> Switch/1
  Switch/1 -> Demux/1
  Demux/1 -> Tm_R (TC)/1
  Demux/2 -> Tm_L (TC)/1

== system TV_full_CARSIM_24b/Traction Control/Trcation Control Algorithm/Low Level TC/excess slip switch ==
  slip_L : Inport
  slip_R : Inport  Port=2
  Constant : Constant
  Constant2 : Constant  Value=0
  Max : MinMax  Function=max  Inputs=2
  Switch1 : Switch  Criteria=u2 > Threshold  Threshold=s_desired  SaturateOnIntegerOverflow=off  InputSameDT=off
  on/off : Outport
  slip : Outport  Port=2
  wires:
  slip_L/1 -> Max/1
  slip_R/1 -> Max/2
  Switch1/1 -> on/off/1
  Max/1 -> slip/1, Switch1/2
  Constant2/1 -> Switch1/3
  Constant/1 -> Switch1/1

== system TV_full_CARSIM_24b/Torque Vectoring/Torque Vectoring Algorithm/Torque Distribution Center/Torque Request Doesn't Surpass T_max/+M_yaw ==
  delta T : Inport
  Torque Requested : Inport  Port=2
  Enable : EnablePort  StatesWhenEnabling=reset
  Abs : Abs  SaturateOnIntegerOverflow=off
  Add : Sum
  Gain : Gain  Gain=0.5
  Subtract : Sum  Inputs=+-
  "T_m, L" : Outport
  T_m,R : Outport  Port=2
  wires:
  delta T/1 -> Abs/1
  Abs/1 -> Gain/1
  Gain/1 -> Add/2, Subtract/2
  Torque Requested/1 -> Subtract/1, Add/1
  Subtract/1 -> "T_m, L"/1
  Add/1 -> T_m,R/1

== system TV_full_CARSIM_24b/Torque Vectoring/Torque Vectoring Algorithm/Torque Distribution Center/Torque Request Doesn't Surpass T_max/-M_yaw ==
  delta T : Inport
  Torque Requested : Inport  Port=2
  Enable : EnablePort  StatesWhenEnabling=reset
  Abs : Abs  SaturateOnIntegerOverflow=off
  Add : Sum
  Gain : Gain  Gain=0.5
  Subtract : Sum  Inputs=+-
  "T_m, L" : Outport
  T_m,R : Outport  Port=2
  wires:
  Torque Requested/1 -> Subtract/1, Add/1
  Abs/1 -> Gain/1
  Gain/1 -> Add/2, Subtract/2
  delta T/1 -> Abs/1
  Subtract/1 -> T_m,R/1
  Add/1 -> "T_m, L"/1

== system TV_full_CARSIM_24b/Torque Vectoring/Torque Vectoring Algorithm/Torque Distribution Center/Torque Request Surpasses T_max/+M_yaw ==
  delta T : Inport
  Torque Requested : Inport  Port=2
  "T_m, max" : Inport  Port=3
  Enable : EnablePort  StatesWhenEnabling=reset
  Abs : Abs  SaturateOnIntegerOverflow=off
  Subtract : Sum  Inputs=+-
  Subtract1 : Sum  Inputs=+-
  Subtract2 : Sum  Inputs=-+
  "T_m, L" : Outport
  T_m,R : Outport  Port=2
  wires:
  "T_m, max"/1 -> T_m,R/1, Subtract/1
  delta T/1 -> Abs/1
  Abs/1 -> Subtract1/1
  Torque Requested/1 -> Subtract2/2, Subtract/2
  Subtract/1 -> Subtract1/2
  Subtract1/1 -> Subtract2/1
  Subtract2/1 -> "T_m, L"/1

== system TV_full_CARSIM_24b/Torque Vectoring/Torque Vectoring Algorithm/Torque Distribution Center/Torque Request Surpasses T_max/-M_yaw ==
  delta T : Inport
  Torque Requested : Inport  Port=2
  "T_m, max" : Inport  Port=3
  Enable : EnablePort  StatesWhenEnabling=reset
  Abs : Abs  SaturateOnIntegerOverflow=off
  Subtract : Sum  Inputs=+-
  Subtract1 : Sum  Inputs=+-
  Subtract2 : Sum  Inputs=-+
  "T_m, L" : Outport
  T_m,R : Outport  Port=2
  wires:
  Torque Requested/1 -> Subtract2/2, Subtract/2
  "T_m, max"/1 -> "T_m, L"/1, Subtract/1
  Subtract/1 -> Subtract1/2
  delta T/1 -> Abs/1
  Subtract1/1 -> Subtract2/1
  Abs/1 -> Subtract1/1
  Subtract2/1 -> T_m,R/1

== system TV_full_CARSIM_24b/Traction Control/Trcation Control Algorithm/Low Level TC/Torque Reduction Algorithm/Left Turn ==
  delta Tmax TC : Inport
  Tm_R : Inport  Port=2
  L_ratio : Inport  Port=3
  Enable : EnablePort
  Constant : Constant
  Divide : Product  Inputs=*/
  Saturation : Saturate  UpperLimit=inf  LowerLimit=0.001
  Subtract : Sum  Inputs=+-
  Sum : Sum  Inputs=|+-
  Tm_R (TC) : Outport
  Tm_L (TC) : Outport  Port=2
  wires:
  Tm_R/1 -> Sum/1
  delta Tmax TC/1 -> Sum/2
  Constant/1 -> Subtract/1
  L_ratio/1 -> Subtract/2
  Sum/1 -> Divide/1, Tm_R (TC)/1
  Subtract/1 -> Saturation/1
  Saturation/1 -> Divide/2
  Divide/1 -> Tm_L (TC)/1

== system TV_full_CARSIM_24b/Traction Control/Trcation Control Algorithm/Low Level TC/Torque Reduction Algorithm/Right Turn ==
  delta Tmax TC : Inport
  Tm_L : Inport  Port=2
  R_ratio : Inport  Port=3
  Enable : EnablePort
  Constant : Constant
  Divide : Product  Inputs=*/
  Saturation : Saturate  UpperLimit=inf  LowerLimit=0.001
  Subtract : Sum  Inputs=+-
  Sum : Sum  Inputs=|+-
  Tm_R (TC) : Outport
  Tm_L (TC) : Outport  Port=2
  wires:
  Sum/1 -> Divide/1, Tm_L (TC)/1
  delta Tmax TC/1 -> Sum/2
  R_ratio/1 -> Subtract/2
  Saturation/1 -> Divide/2
  Constant/1 -> Subtract/1
  Subtract/1 -> Saturation/1
  Divide/1 -> Tm_R (TC)/1
  Tm_L/1 -> Sum/1

== system TV_full_CARSIM_24b/Traction Control/Trcation Control Algorithm/Low Level TC/Torque Reduction Algorithm/TC Feedback ==
  slip : Inport
  Constant : Constant  Value=s_desired
  PID Controller : slpidlib/PID Controller  Controller=PID  Form=Parallel  TimeDomain=Continuous-time  UseExternalTs=off  SampleTime=-1  IntegratorMethod=Forward Euler  FilterMethod=Forward Euler  ControllerParametersSource=internal  P=1  I=1  UseKiTs=off  D=0  UseExternalDerivativeSource=off  N=100  UseFilter=on  TunerSelectOption=Transfer Function Based (PID Tuner App)  InitialConditionSource=internal  InitialConditionForIntegrator=0  InitialConditionForFilter=0  DifferentiatorICPrevScaledInput=0  ExternalReset=none  TrackingMode=off  Kt=1  LimitOutput=off  SatLimitsSource=internal  UpperSaturationLimit=inf  LowerSaturationLimit=-inf  LinearizeAsGain=on  AntiWindupMode=none  Kb=1  LimitIntegrator=off  UpperIntegratorSaturationLimit=inf  LowerIntegratorSaturationLimit=-inf  POutMin=[]  POutMax=[]  IOutMin=[]  IOutMax=[]  DOutMin=[]  DOutMax=[]  NOutMin=[]  NOutMax=[]  SumOutMin=[]  SumOutMax=[]  SaturationOutMin=[]  SaturationOutMax=[]  PParamMin=[]  PParamMax=[]  IParamMin=[]  IParamMax=[]  DParamMin=[]  DParamMax=[]  NParamMin=[]  NParamMax=[]  KbParamMin=[]  KbParamMax=[]  KtParamMin=[]  KtParamMax=[]  KbOutMin=[]  KbOutMax=[]  KtOutMin=[]  KtOutMax=[]  IntegratorOutMin=[]  IntegratorOutMax=[]  FilterOutMin=[]  FilterOutMax=[]  SumI1OutMin=[]  SumI1OutMax=[]  SumI2OutMin=[]  SumI2OutMax=[]  SumI3OutMin=[]  SumI3OutMax=[]  SumI4OutMin=[]  SumI4OutMax=[]  SumDOutMin=[]  SumDOutMax=[]  DifferentiatorOutMin=[]  DifferentiatorOutMax=[]  FilterDiffOutCoefMin=[]  FilterDiffOutCoefMax=[]  ReciprocalOutMin=[]  ReciprocalOutMax=[]  SumDenOutMin=[]  SumDenOutMax=[]  SumNumOutMin=[]  SumNumOutMax=[]  DivideOutMin=[]  DivideOutMax=[]  UdiffTsProdOutMin=[]  UdiffTsProdOutMax=[]  NTsProdOutMin=[]  NTsProdOutMax=[]  UintegralTsProdOutMin=[]  UintegralTsProdOutMax=[]  UngainTsProdOutMin=[]  UngainTsProdOutMax=[]  ClampingZeroOutDataTypeStr=Inherit: Inherit via back propagation  ClampingZeroOutMin=[]  ClampingZeroOutMax=[]  FilterDenConstantOutDataTypeStr=Inherit: Inherit via back propagation  FilterDenConstantOutMin=[]  FilterDenConstantOutMax=[]  PCopyOutDataTypeStr=Inherit: Inherit via back propagation  PCopyOutMin=[]  PCopyOutMax=[]  NCopyOutDataTypeStr=Inherit: Inherit via back propagation  NCopyOutMin=[]  NCopyOutMax=[]  IntegratorContinuousStateAttributes=''  IntegratorStateMustResolveToSignalObject=off  IntegratorRTWStateStorageClass=Auto  FilterContinuousStateAttributes=''  FilterStateMustResolveToSignalObject=off  FilterRTWStateStorageClass=Auto  ParallelPVariant=InternalParameters  IdealPVariant=Disabled  IVariant=InternalParameters  DVariant=InternalParameters  IntegratorVariant=Continuous  SatVariant=Disabled  AWVariant=Passthrough  PCopyVariant=Disabled  TRVariant=Disabled  FdbkBlocksVariant=Forward  IdealPFdbkVariant=Disabled  SatFdbkVariant=Disabled  DerivativeFilterVariant=ContFilter  NVariant=InternalParameters  NCopyVariant=Disabled  FilterICVariant=InternalICsFilter  IntegratorICVariant=InternalICs  ExternalResetVariant=Disabled  TRSumVariant=Passthrough  SumFdbkVariant=Disabled  SumVariant=Sum_PID  TsampFilterVariant=InternalTs  TsampNgainVariant=Passthrough  TsampIntegralVariant=Disabled_SignalSpec  ExternalSaturationOutDataTypeStr=Inherit: Same as second input  DerivativeSourceVariant=ErrorSignal  PreIntVariant=InternalPreInt
  Saturation : Saturate  UpperLimit=Tmax  LowerLimit=0
  Sum : Sum  Inputs=|+-
  delta Tmax TC : Outport
  wires:
  Constant/1 -> Sum/1
  Sum/1 -> PID Controller/1
  PID Controller/1 -> Saturation/1
  slip/1 -> Sum/2
  Saturation/1 -> delta Tmax TC/1

== system TV_full_CARSIM_24b/Traction Control/Trcation Control Algorithm/Low Level TC/Torque Reduction Algorithm/Torque Ratio Calculations ==
  Tm_L : Inport
  Tm_R : Inport  Port=2
  Divide : Product  Inputs=*/
  Divide1 : Product  Inputs=*/
  Saturation : Saturate  UpperLimit=inf  LowerLimit=0.001
  Sum : Sum  Inputs=|++
  L_ratio : Outport
  R_ratio : Outport  Port=2
  wires:
  Tm_L/1 -> Divide/1, Sum/1
  Tm_R/1 -> Sum/2, Divide1/1
  Sum/1 -> Saturation/1
  Saturation/1 -> Divide1/2, Divide/2
  Divide/1 -> L_ratio/1
  Divide1/1 -> R_ratio/1
